simulink library "monroe_library"  (R2012b)
settings: Solver=ode45  StartTime=0.0  StopTime=10.0  RelTol=1e-3
values from neighbouring files (symbols this model uses):
  input_bit_width = ', num2str(input_bit_width))    [fft_direct_draw.m]
undefined symbols (not defined in the file or in its folder): gcbh, xlBlockLoadCallback
libraries: xbsIndex_r4 x1880, monroe_library x159, casper_library x13, xps_library x1
(part 41 of 43)

== system monroe_library/unscr_tail/mirror_spectrum/Subsystem ==
  In1 : Inport
  In3 : Inport  Port=2
  In4 : Inport  Port=3
  Delay11 : S-Function  LoadFcn=xlBlockLoadCallback(gcbh);  FunctionName=sysgen  Parameters=ptable_  EnableBusSupport=off  mask(Xilinx Delay Block){infoedit=Hardware notes: A delay line is a chain, each link of which is an SRL16 followed by a flip-flop., en_sgadvanced=, en=off, latency=1, dbl_ovrd_sgadvanced=, dbl_ovrd=off, reg_retiming_sgadvanced=, reg_retiming=off, xl_use_area_sgadvanced=, xl_use_area=off, xl_area=[0,0,0,0,0,0,0], has_advanced_control=0, sggui_pos=-1,-1,-1,-1, block_type=delay, block_version=, sg_icon_stat=25,28,1,1,white,blue,0,07b98262,right,,[ ],[ ], sg_mask_display=|, sg_list_contents=, sg_blockgui_xml=}
      mask sg_mask_display=|
      | fprintf('','COMMENT: begin icon graphics');
      | patch([0 25 25 0 0 ],[0 0 28 28 0 ],[0.77 0.82 0.91 ]);
      | plot([0 25 25 0 0 ],[0 0 28 28 0 ]);
      | patch([5.325 9.66 12.66 15.66 18.66 12.66 8.325 5.325 ],[17.33 17.33 20.33 17.33 20.33 20.33 20.33 17.33 ],[1 1 1 ]);
      | patch([8.325 12.66 9.66 5.325 8.325 ],[14.33 14.33 17.33 17.33 14.33 ],[0.931 0.946 0.973 ]);
      | patch([5.325 9.66 12.66 8.325 5.325 ],[11.33 11.33 14.33 14.33 11.33 ],[1 1 1 ]);
      | patch([8.325 18.66 15.66 12.66 9.66 5.325 8.325 ],[8.33 8.33 11.33 8.33 11.33 11.33 8.33 ],[0.931 0.946 0.973 ]);
      | fprintf('','COMMENT: end icon graphics');
      | fprintf('','COMMENT: begin icon text');
      |
      |
      | color('black');disp('z^{-1}','texmode','on');
      | fprintf('','COMMENT: end icon text');
      mask prompts: infoedit ""; en_sgadvanced ""; en "Provide enable port"; dbl_ovrd_sgadvanced ""; dbl_ovrd "Override with doubles"; reg_retiming_sgadvanced ""; reg_retiming "Implement using behavioral HDL."; xl_use_area_sgadvanced ""; xl_use_area "Define FPGA area for resource estimation"; xl_area "FPGA area [slices, FFs, BRAMs, LUTs, IOBs, emb. mults, TBUFs]"; has_advanced_control ""; sggui_pos ""; block_type ""; block_version ""; sg_icon_stat ""; sg_mask_display ""; sg_list_contents ""; sg_blockgui_xml ""
      mask help: Hardware notes: A delay line is a chain, each link of which is an SRL16 followed by a flip-flop.
      mask init: same as monroe_library/counter_limited_fast/Delay1
      settings: CopyFcn=xlBlockMoveCallback(gcbh);  DeleteFcn=xlDestroyGui(gcbh);  ModelCloseFcn=xlDestroyGui(gcbh);  PreSaveFcn=xlBlockPreSaveCallback(gcbh);  PostSaveFcn=xlBlockPostSaveCallback(gcbh);  DestroyFcn=xlDestroyGui(gcbh);  OpenFcn=xlOpenGui(gcbh, 'delay_gui.xml', @xlmagicenablement, -1)  CloseFcn=xlDestroyGui(gcbh);  MoveFcn=xlBlockMoveCallback(gcbh);
      mask Help: eval('');xlDoc('-book','sysgen','-topic','Delay');
      mask Display:
      | fprintf('','COMMENT: begin icon graphics');
      | patch([0 25 25 0 0 ],[0 0 28 28 0 ],[0.77 0.82 0.91 ]);
      | plot([0 25 25 0 0 ],[0 0 28 28 0 ]);
      | patch([5.325 9.66 12.66 15.66 18.66 12.66 8.325 5.325 ],[17.33 17.33 20.33 17.33 20.33 20.33 20.33 17.33 ],[1 1 1 ]);
      | patch([8.325 12.66 9.66 5.325 8.325 ],[14.33 14.33 17.33 17.33 14.33 ],[0.931 0.946 0.973 ]);
      | patch([5.325 9.66 12.66 8.325 5.325 ],[11.33 11.33 14.33 14.33 11.33 ],[1 1 1 ]);
      | patch([8.325 18.66 15.66 12.66 9.66 5.325 8.325 ],[8.33 8.33 11.33 8.33 11.33 11.33 8.33 ],[0.931 0.946 0.973 ]);
      | fprintf('','COMMENT: end icon graphics');
      | fprintf('','COMMENT: begin icon text');
      | 
      | 
      | color('black');disp('z^{-1}','texmode','on');
      | fprintf('','COMMENT: end icon text');
  Delay7 : xbsIndex_r4/Delay  en=off  latency=1  dbl_ovrd=off  reg_retiming=off  block_type=delay
  Mux4 : S-Function  LoadFcn=xlBlockLoadCallback(gcbh);  FunctionName=sysgen  Parameters=ptable_  EnableBusSupport=off  mask(Xilinx Bus Multiplexer Block){inputs_sgadvanced=, inputs=2, en_sgadvanced=, en=off, latency=0, precision_sgadvanced=, precision=Full, arith_type_sgadvanced=, arith_type=Signed  (2's comp), n_bits=8, bin_pt=2, quantization_sgadvanced=, quantization=Truncate, overflow_sgadvanced=, overflow=Wrap, dbl_ovrd_sgadvanced=, dbl_ovrd=off, xl_use_area_sgadvanced=, xl_use_area=off, xl_area=[0,0,0,0,0,0,0], infoedit=, has_advanced_control=0, sggui_pos=-1,-1,-1,-1, block_type=mux, block_version=, sg_icon_stat=45,104,3,1,white,blue,3,eb98d690,right,,[ ],[ ], sg_mask_display=|, sg_list_contents=, sg_blockgui_xml=}
      mask sg_mask_display=|
      | fprintf('','COMMENT: begin icon graphics');
      | patch([0 45 45 0 0 ],[0 14.8571 89.1429 104 0 ],[0.77 0.82 0.91 ]);
      | plot([0 45 45 0 0 ],[0 14.8571 89.1429 104 0 ]);
      | patch([8.65 17.32 23.32 29.32 35.32 23.32 14.65 8.65 ],[58.66 58.66 64.66 58.66 64.66 64.66 64.66 58.66 ],[1 1 1 ]);
      | patch([14.65 23.32 17.32 8.65 14.65 ],[52.66 52.66 58.66 58.66 52.66 ],[0.931 0.946 0.973 ]);
      | patch([8.65 17.32 23.32 14.65 8.65 ],[46.66 46.66 52.66 52.66 46.66 ],[1 1 1 ]);
      | patch([14.65 35.32 29.32 23.32 17.32 8.65 14.65 ],[40.66 40.66 46.66 40.66 46.66 46.66 40.66 ],[0.931 0.946 0.973 ]);
      | fprintf('','COMMENT: end icon graphics');
      | fprintf('','COMMENT: begin icon text');
      | color('black');port_label('input',1,'sel');
      | color('black');port_label('input',2,'d0');
      | color('black');port_label('input',3,'d1');
      |
      | color('black');disp('\bf{}','texmode','on');
      | fprintf('','COMMENT: end icon text');
      mask prompts: inputs_sgadvanced ""; inputs "Number of inputs"; en_sgadvanced ""; en "Provide enable port"; precision_sgadvanced ""; arith_type_sgadvanced ""; arith_type "Output type"; n_bits "Number of bits"; bin_pt "Binary point"; quantization_sgadvanced ""; overflow_sgadvanced ""; dbl_ovrd_sgadvanced ""; dbl_ovrd "Override with doubles"; xl_use_area_sgadvanced ""; xl_use_area "Define FPGA area for resource estimation"; xl_area "FPGA area [slices, FFs, BRAMs, LUTs, IOBs, emb. mults, TBUFs]"; infoedit ""; has_advanced_control ""; sggui_pos ""; block_type ""; block_version ""; sg_icon_stat ""; sg_mask_display ""; sg_list_contents ""; sg_blockgui_xml ""
      mask help: Xilinx Bus Multiplexer
      mask init:
      | try
      |   tmp_gcb = gcb;
      |   tmp_gcbh = gcbh;
      |   if (strcmp('SysGenIndex',get_param(bdroot(tmp_gcbh),'tag')) && ~isempty(regexp(bdroot(tmp_gcb), '^xbs', 'once')))
      |     return;
      |   end;
      |   xlMungeMaskParams;
      |   block_config = 'sysgen_blockset:Mux_config';
      | 
      |   block_type='mux';
      | 
      |   serialized_declarations = '{''arith_type''=>''Int'',''bin_pt''=>''Int'',''dbl_ovrd''=>''Int'',''en''=>''Int'',''inputs''=>''Int'',''latency''=>''Int'',''n_bits''=>''Int'',''overflow''=>''Int'',''period''=>''Double'',''precision''=>''Int'',''quantization''=>''Int'',''sim_engine''=>''Int'',''sysgen_root''=>''String'',''block_type''=>''String''}';
      |   xlmux_init();
      |   ptable_ = xlblockprep(get_param(tmp_gcb, 'MaskWSVariables'));
      |   try
      |     xlBlockMoveCallback(tmp_gcbh);
      |   catch 
      |      clear global xl_updateicon_recursion_guard;
      |   end;
      | catch
      |   global dbgsysgen;
      |   if(~isempty(dbgsysgen) && dbgsysgen)
      |     e = regexprep(lasterr, '\n', '\nError: ');
      |     disp(['Error: While running MaskInit code on block ' tmp_gcb ': ' e]);
      |     error(e);
      |   end
      | end
      settings: CopyFcn=xlBlockMoveCallback(gcbh);  DeleteFcn=xlDestroyGui(gcbh);  ModelCloseFcn=xlDestroyGui(gcbh);  PreSaveFcn=xlBlockPreSaveCallback(gcbh);  PostSaveFcn=xlBlockPostSaveCallback(gcbh);  DestroyFcn=xlDestroyGui(gcbh);  OpenFcn=xlOpenGui(gcbh, 'mux_gui.xml', @muxenablement, -1)  CloseFcn=xlDestroyGui(gcbh);  MoveFcn=xlBlockMoveCallback(gcbh);
      mask Help: eval('');xlDoc('-book','sysgen','-topic','Mux');
      mask TypeOptions inputs: 2 | 3 | 4 | 5 | 6 | 7 | 8 | 9 | 10 | 11 | 12 | 13 | 14 | 15 | 16 | 17 | 18 | 19 | 20 | 21 | 22 | 23 | 24 | 25 | 26 | 27 | 28 | 29 | 30 | 31 | 32
      mask TypeOptions precision: Full | User Defined
      mask TypeOptions arith_type: Signed  (2's comp) | Unsigned
      mask TypeOptions quantization: Truncate | Round  (unbiased: +/- Inf)
      mask TypeOptions overflow: Wrap | Saturate | Flag as error
      mask Display:
      | fprintf('','COMMENT: begin icon graphics');
      | patch([0 45 45 0 0 ],[0 14.8571 89.1429 104 0 ],[0.77 0.82 0.91 ]);
      | plot([0 45 45 0 0 ],[0 14.8571 89.1429 104 0 ]);
      | patch([8.65 17.32 23.32 29.32 35.32 23.32 14.65 8.65 ],[58.66 58.66 64.66 58.66 64.66 64.66 64.66 58.66 ],[1 1 1 ]);
      | patch([14.65 23.32 17.32 8.65 14.65 ],[52.66 52.66 58.66 58.66 52.66 ],[0.931 0.946 0.973 ]);
      | patch([8.65 17.32 23.32 14.65 8.65 ],[46.66 46.66 52.66 52.66 46.66 ],[1 1 1 ]);
      | patch([14.65 35.32 29.32 23.32 17.32 8.65 14.65 ],[40.66 40.66 46.66 40.66 46.66 46.66 40.66 ],[0.931 0.946 0.973 ]);
      | fprintf('','COMMENT: end icon graphics');
      | fprintf('','COMMENT: begin icon text');
      | color('black');port_label('input',1,'sel');
      | color('black');port_label('input',2,'d0');
      | color('black');port_label('input',3,'d1');
      | 
      | color('black');disp('\bf{}','texmode','on');
      | fprintf('','COMMENT: end icon text');
  Mux5 : S-Function  LoadFcn=xlBlockLoadCallback(gcbh);  FunctionName=sysgen  Parameters=ptable_  EnableBusSupport=off  mask(Xilinx Bus Multiplexer Block){inputs_sgadvanced=, inputs=2, en_sgadvanced=, en=off, latency=0, precision_sgadvanced=, precision=Full, arith_type_sgadvanced=, arith_type=Signed  (2's comp), n_bits=8, bin_pt=2, quantization_sgadvanced=, quantization=Truncate, overflow_sgadvanced=, overflow=Wrap, dbl_ovrd_sgadvanced=, dbl_ovrd=off, xl_use_area_sgadvanced=, xl_use_area=off, xl_area=[0,0,0,0,0,0,0], infoedit=, has_advanced_control=0, sggui_pos=-1,-1,-1,-1, block_type=mux, block_version=, sg_icon_stat=45,104,3,1,white,blue,3,eb98d690,right,,[ ],[ ], sg_mask_display=|, sg_list_contents=, sg_blockgui_xml=}
      mask sg_mask_display=|
      | fprintf('','COMMENT: begin icon graphics');
      | patch([0 45 45 0 0 ],[0 14.8571 89.1429 104 0 ],[0.77 0.82 0.91 ]);
      | plot([0 45 45 0 0 ],[0 14.8571 89.1429 104 0 ]);
      | patch([8.65 17.32 23.32 29.32 35.32 23.32 14.65 8.65 ],[58.66 58.66 64.66 58.66 64.66 64.66 64.66 58.66 ],[1 1 1 ]);
      | patch([14.65 23.32 17.32 8.65 14.65 ],[52.66 52.66 58.66 58.66 52.66 ],[0.931 0.946 0.973 ]);
      | patch([8.65 17.32 23.32 14.65 8.65 ],[46.66 46.66 52.66 52.66 46.66 ],[1 1 1 ]);
      | patch([14.65 35.32 29.32 23.32 17.32 8.65 14.65 ],[40.66 40.66 46.66 40.66 46.66 46.66 40.66 ],[0.931 0.946 0.973 ]);
      | fprintf('','COMMENT: end icon graphics');
      | fprintf('','COMMENT: begin icon text');
      | color('black');port_label('input',1,'sel');
      | color('black');port_label('input',2,'d0');
      | color('black');port_label('input',3,'d1');
      |
      | color('black');disp('\bf{}','texmode','on');
      | fprintf('','COMMENT: end icon text');
      mask prompts: inputs_sgadvanced ""; inputs "Number of inputs"; en_sgadvanced ""; en "Provide enable port"; precision_sgadvanced ""; arith_type_sgadvanced ""; arith_type "Output type"; n_bits "Number of bits"; bin_pt "Binary point"; quantization_sgadvanced ""; overflow_sgadvanced ""; dbl_ovrd_sgadvanced ""; dbl_ovrd "Override with doubles"; xl_use_area_sgadvanced ""; xl_use_area "Define FPGA area for resource estimation"; xl_area "FPGA area [slices, FFs, BRAMs, LUTs, IOBs, emb. mults, TBUFs]"; infoedit ""; has_advanced_control ""; sggui_pos ""; block_type ""; block_version ""; sg_icon_stat ""; sg_mask_display ""; sg_list_contents ""; sg_blockgui_xml ""
      mask help: Xilinx Bus Multiplexer
      mask init: same as monroe_library/unscr_tail/mirror_spectrum/Subsystem/Mux4
      settings: CopyFcn=xlBlockMoveCallback(gcbh);  DeleteFcn=xlDestroyGui(gcbh);  ModelCloseFcn=xlDestroyGui(gcbh);  PreSaveFcn=xlBlockPreSaveCallback(gcbh);  PostSaveFcn=xlBlockPostSaveCallback(gcbh);  DestroyFcn=xlDestroyGui(gcbh);  OpenFcn=xlOpenGui(gcbh, 'mux_gui.xml', @muxenablement, -1)  CloseFcn=xlDestroyGui(gcbh);  MoveFcn=xlBlockMoveCallback(gcbh);
      mask Help: eval('');xlDoc('-book','sysgen','-topic','Mux');
      mask TypeOptions inputs: 2 | 3 | 4 | 5 | 6 | 7 | 8 | 9 | 10 | 11 | 12 | 13 | 14 | 15 | 16 | 17 | 18 | 19 | 20 | 21 | 22 | 23 | 24 | 25 | 26 | 27 | 28 | 29 | 30 | 31 | 32
      mask TypeOptions precision: Full | User Defined
      mask TypeOptions arith_type: Signed  (2's comp) | Unsigned
      mask TypeOptions quantization: Truncate | Round  (unbiased: +/- Inf)
      mask TypeOptions overflow: Wrap | Saturate | Flag as error
      mask Display:
      | fprintf('','COMMENT: begin icon graphics');
      | patch([0 45 45 0 0 ],[0 14.8571 89.1429 104 0 ],[0.77 0.82 0.91 ]);
      | plot([0 45 45 0 0 ],[0 14.8571 89.1429 104 0 ]);
      | patch([8.65 17.32 23.32 29.32 35.32 23.32 14.65 8.65 ],[58.66 58.66 64.66 58.66 64.66 64.66 64.66 58.66 ],[1 1 1 ]);
      | patch([14.65 23.32 17.32 8.65 14.65 ],[52.66 52.66 58.66 58.66 52.66 ],[0.931 0.946 0.973 ]);
      | patch([8.65 17.32 23.32 14.65 8.65 ],[46.66 46.66 52.66 52.66 46.66 ],[1 1 1 ]);
      | patch([14.65 35.32 29.32 23.32 17.32 8.65 14.65 ],[40.66 40.66 46.66 40.66 46.66 46.66 40.66 ],[0.931 0.946 0.973 ]);
      | fprintf('','COMMENT: end icon graphics');
      | fprintf('','COMMENT: begin icon text');
      | color('black');port_label('input',1,'sel');
      | color('black');port_label('input',2,'d0');
      | color('black');port_label('input',3,'d1');
      | 
      | color('black');disp('\bf{}','texmode','on');
      | fprintf('','COMMENT: end icon text');
  cram5 : Subsystem
  uncram5 : monroe_library/unscr_tail/mirror_spectrum/uncram1  SystemSampleTime=-1
  uncram6 : Subsystem
  Out1 : Outport
  wires:
  uncram5/1 -> Mux4/2
  uncram6/1(out0) -> Mux4/3
  uncram5/2 -> Mux5/2
  uncram6/2(out1) -> Mux5/3
  Delay11/1 -> Mux4/1
  Delay7/1 -> Mux5/1
  Mux5/1 -> cram5/2(in1)
  Mux4/1 -> cram5/1(in0)
  In1/1 -> Delay11/1, Delay7/1
  cram5/1(out) -> Out1/1
  In3/1 -> uncram5/1
  In4/1 -> uncram6/1(in)

== system monroe_library/unscr_tail/mirror_spectrum/Subsystem1 ==
  In1 : Inport
  In3 : Inport  Port=2
  In4 : Inport  Port=3
  Delay11 : S-Function  LoadFcn=xlBlockLoadCallback(gcbh);  FunctionName=sysgen  Parameters=ptable_  EnableBusSupport=off  mask(Xilinx Delay Block){infoedit=Hardware notes: A delay line is a chain, each link of which is an SRL16 followed by a flip-flop., en_sgadvanced=, en=off, latency=1, dbl_ovrd_sgadvanced=, dbl_ovrd=off, reg_retiming_sgadvanced=, reg_retiming=off, xl_use_area_sgadvanced=, xl_use_area=off, xl_area=[0,0,0,0,0,0,0], has_advanced_control=0, sggui_pos=-1,-1,-1,-1, block_type=delay, block_version=, sg_icon_stat=25,28,1,1,white,blue,0,07b98262,right,,[ ],[ ], sg_mask_display=|, sg_list_contents=, sg_blockgui_xml=}
      mask sg_mask_display=|
      | fprintf('','COMMENT: begin icon graphics');
      | patch([0 25 25 0 0 ],[0 0 28 28 0 ],[0.77 0.82 0.91 ]);
      | plot([0 25 25 0 0 ],[0 0 28 28 0 ]);
      | patch([5.325 9.66 12.66 15.66 18.66 12.66 8.325 5.325 ],[17.33 17.33 20.33 17.33 20.33 20.33 20.33 17.33 ],[1 1 1 ]);
      | patch([8.325 12.66 9.66 5.325 8.325 ],[14.33 14.33 17.33 17.33 14.33 ],[0.931 0.946 0.973 ]);
      | patch([5.325 9.66 12.66 8.325 5.325 ],[11.33 11.33 14.33 14.33 11.33 ],[1 1 1 ]);
      | patch([8.325 18.66 15.66 12.66 9.66 5.325 8.325 ],[8.33 8.33 11.33 8.33 11.33 11.33 8.33 ],[0.931 0.946 0.973 ]);
      | fprintf('','COMMENT: end icon graphics');
      | fprintf('','COMMENT: begin icon text');
      |
      |
      | color('black');disp('z^{-1}','texmode','on');
      | fprintf('','COMMENT: end icon text');
      mask prompts: infoedit ""; en_sgadvanced ""; en "Provide enable port"; dbl_ovrd_sgadvanced ""; dbl_ovrd "Override with doubles"; reg_retiming_sgadvanced ""; reg_retiming "Implement using behavioral HDL."; xl_use_area_sgadvanced ""; xl_use_area "Define FPGA area for resource estimation"; xl_area "FPGA area [slices, FFs, BRAMs, LUTs, IOBs, emb. mults, TBUFs]"; has_advanced_control ""; sggui_pos ""; block_type ""; block_version ""; sg_icon_stat ""; sg_mask_display ""; sg_list_contents ""; sg_blockgui_xml ""
      mask help: Hardware notes: A delay line is a chain, each link of which is an SRL16 followed by a flip-flop.
      mask init: same as monroe_library/counter_limited_fast/Delay1
      settings: CopyFcn=xlBlockMoveCallback(gcbh);  DeleteFcn=xlDestroyGui(gcbh);  ModelCloseFcn=xlDestroyGui(gcbh);  PreSaveFcn=xlBlockPreSaveCallback(gcbh);  PostSaveFcn=xlBlockPostSaveCallback(gcbh);  DestroyFcn=xlDestroyGui(gcbh);  OpenFcn=xlOpenGui(gcbh, 'delay_gui.xml', @xlmagicenablement, -1)  CloseFcn=xlDestroyGui(gcbh);  MoveFcn=xlBlockMoveCallback(gcbh);
      mask Help: eval('');xlDoc('-book','sysgen','-topic','Delay');
      mask Display:
      | fprintf('','COMMENT: begin icon graphics');
      | patch([0 25 25 0 0 ],[0 0 28 28 0 ],[0.77 0.82 0.91 ]);
      | plot([0 25 25 0 0 ],[0 0 28 28 0 ]);
      | patch([5.325 9.66 12.66 15.66 18.66 12.66 8.325 5.325 ],[17.33 17.33 20.33 17.33 20.33 20.33 20.33 17.33 ],[1 1 1 ]);
      | patch([8.325 12.66 9.66 5.325 8.325 ],[14.33 14.33 17.33 17.33 14.33 ],[0.931 0.946 0.973 ]);
      | patch([5.325 9.66 12.66 8.325 5.325 ],[11.33 11.33 14.33 14.33 11.33 ],[1 1 1 ]);
      | patch([8.325 18.66 15.66 12.66 9.66 5.325 8.325 ],[8.33 8.33 11.33 8.33 11.33 11.33 8.33 ],[0.931 0.946 0.973 ]);
      | fprintf('','COMMENT: end icon graphics');
      | fprintf('','COMMENT: begin icon text');
      | 
      | 
      | color('black');disp('z^{-1}','texmode','on');
      | fprintf('','COMMENT: end icon text');
  Delay7 : xbsIndex_r4/Delay  en=off  latency=1  dbl_ovrd=off  reg_retiming=off  block_type=delay
  Mux4 : S-Function  LoadFcn=xlBlockLoadCallback(gcbh);  FunctionName=sysgen  Parameters=ptable_  EnableBusSupport=off  mask(Xilinx Bus Multiplexer Block){inputs_sgadvanced=, inputs=2, en_sgadvanced=, en=off, latency=0, precision_sgadvanced=, precision=Full, arith_type_sgadvanced=, arith_type=Signed  (2's comp), n_bits=8, bin_pt=2, quantization_sgadvanced=, quantization=Truncate, overflow_sgadvanced=, overflow=Wrap, dbl_ovrd_sgadvanced=, dbl_ovrd=off, xl_use_area_sgadvanced=, xl_use_area=off, xl_area=[0,0,0,0,0,0,0], infoedit=, has_advanced_control=0, sggui_pos=-1,-1,-1,-1, block_type=mux, block_version=, sg_icon_stat=45,104,3,1,white,blue,3,eb98d690,right,,[ ],[ ], sg_mask_display=|, sg_list_contents=, sg_blockgui_xml=}
      mask sg_mask_display=|
      | fprintf('','COMMENT: begin icon graphics');
      | patch([0 45 45 0 0 ],[0 14.8571 89.1429 104 0 ],[0.77 0.82 0.91 ]);
      | plot([0 45 45 0 0 ],[0 14.8571 89.1429 104 0 ]);
      | patch([8.65 17.32 23.32 29.32 35.32 23.32 14.65 8.65 ],[58.66 58.66 64.66 58.66 64.66 64.66 64.66 58.66 ],[1 1 1 ]);
      | patch([14.65 23.32 17.32 8.65 14.65 ],[52.66 52.66 58.66 58.66 52.66 ],[0.931 0.946 0.973 ]);
      | patch([8.65 17.32 23.32 14.65 8.65 ],[46.66 46.66 52.66 52.66 46.66 ],[1 1 1 ]);
      | patch([14.65 35.32 29.32 23.32 17.32 8.65 14.65 ],[40.66 40.66 46.66 40.66 46.66 46.66 40.66 ],[0.931 0.946 0.973 ]);
      | fprintf('','COMMENT: end icon graphics');
      | fprintf('','COMMENT: begin icon text');
      | color('black');port_label('input',1,'sel');
      | color('black');port_label('input',2,'d0');
      | color('black');port_label('input',3,'d1');
      |
      | color('black');disp('\bf{}','texmode','on');
      | fprintf('','COMMENT: end icon text');
      mask prompts: inputs_sgadvanced ""; inputs "Number of inputs"; en_sgadvanced ""; en "Provide enable port"; precision_sgadvanced ""; arith_type_sgadvanced ""; arith_type "Output type"; n_bits "Number of bits"; bin_pt "Binary point"; quantization_sgadvanced ""; overflow_sgadvanced ""; dbl_ovrd_sgadvanced ""; dbl_ovrd "Override with doubles"; xl_use_area_sgadvanced ""; xl_use_area "Define FPGA area for resource estimation"; xl_area "FPGA area [slices, FFs, BRAMs, LUTs, IOBs, emb. mults, TBUFs]"; infoedit ""; has_advanced_control ""; sggui_pos ""; block_type ""; block_version ""; sg_icon_stat ""; sg_mask_display ""; sg_list_contents ""; sg_blockgui_xml ""
      mask help: Xilinx Bus Multiplexer
      mask init: same as monroe_library/unscr_tail/mirror_spectrum/Subsystem/Mux4
      settings: CopyFcn=xlBlockMoveCallback(gcbh);  DeleteFcn=xlDestroyGui(gcbh);  ModelCloseFcn=xlDestroyGui(gcbh);  PreSaveFcn=xlBlockPreSaveCallback(gcbh);  PostSaveFcn=xlBlockPostSaveCallback(gcbh);  DestroyFcn=xlDestroyGui(gcbh);  OpenFcn=xlOpenGui(gcbh, 'mux_gui.xml', @muxenablement, -1)  CloseFcn=xlDestroyGui(gcbh);  MoveFcn=xlBlockMoveCallback(gcbh);
      mask Help: eval('');xlDoc('-book','sysgen','-topic','Mux');
      mask TypeOptions inputs: 2 | 3 | 4 | 5 | 6 | 7 | 8 | 9 | 10 | 11 | 12 | 13 | 14 | 15 | 16 | 17 | 18 | 19 | 20 | 21 | 22 | 23 | 24 | 25 | 26 | 27 | 28 | 29 | 30 | 31 | 32
      mask TypeOptions precision: Full | User Defined
      mask TypeOptions arith_type: Signed  (2's comp) | Unsigned
      mask TypeOptions quantization: Truncate | Round  (unbiased: +/- Inf)
      mask TypeOptions overflow: Wrap | Saturate | Flag as error
      mask Display:
      | fprintf('','COMMENT: begin icon graphics');
      | patch([0 45 45 0 0 ],[0 14.8571 89.1429 104 0 ],[0.77 0.82 0.91 ]);
      | plot([0 45 45 0 0 ],[0 14.8571 89.1429 104 0 ]);
      | patch([8.65 17.32 23.32 29.32 35.32 23.32 14.65 8.65 ],[58.66 58.66 64.66 58.66 64.66 64.66 64.66 58.66 ],[1 1 1 ]);
      | patch([14.65 23.32 17.32 8.65 14.65 ],[52.66 52.66 58.66 58.66 52.66 ],[0.931 0.946 0.973 ]);
      | patch([8.65 17.32 23.32 14.65 8.65 ],[46.66 46.66 52.66 52.66 46.66 ],[1 1 1 ]);
      | patch([14.65 35.32 29.32 23.32 17.32 8.65 14.65 ],[40.66 40.66 46.66 40.66 46.66 46.66 40.66 ],[0.931 0.946 0.973 ]);
      | fprintf('','COMMENT: end icon graphics');
      | fprintf('','COMMENT: begin icon text');
      | color('black');port_label('input',1,'sel');
      | color('black');port_label('input',2,'d0');
      | color('black');port_label('input',3,'d1');
      | 
      | color('black');disp('\bf{}','texmode','on');
      | fprintf('','COMMENT: end icon text');
  Mux5 : S-Function  LoadFcn=xlBlockLoadCallback(gcbh);  FunctionName=sysgen  Parameters=ptable_  EnableBusSupport=off  mask(Xilinx Bus Multiplexer Block){inputs_sgadvanced=, inputs=2, en_sgadvanced=, en=off, latency=0, precision_sgadvanced=, precision=Full, arith_type_sgadvanced=, arith_type=Signed  (2's comp), n_bits=8, bin_pt=2, quantization_sgadvanced=, quantization=Truncate, overflow_sgadvanced=, overflow=Wrap, dbl_ovrd_sgadvanced=, dbl_ovrd=off, xl_use_area_sgadvanced=, xl_use_area=off, xl_area=[0,0,0,0,0,0,0], infoedit=, has_advanced_control=0, sggui_pos=-1,-1,-1,-1, block_type=mux, block_version=, sg_icon_stat=45,104,3,1,white,blue,3,eb98d690,right,,[ ],[ ], sg_mask_display=|, sg_list_contents=, sg_blockgui_xml=}
      mask sg_mask_display=|
      | fprintf('','COMMENT: begin icon graphics');
      | patch([0 45 45 0 0 ],[0 14.8571 89.1429 104 0 ],[0.77 0.82 0.91 ]);
      | plot([0 45 45 0 0 ],[0 14.8571 89.1429 104 0 ]);
      | patch([8.65 17.32 23.32 29.32 35.32 23.32 14.65 8.65 ],[58.66 58.66 64.66 58.66 64.66 64.66 64.66 58.66 ],[1 1 1 ]);
      | patch([14.65 23.32 17.32 8.65 14.65 ],[52.66 52.66 58.66 58.66 52.66 ],[0.931 0.946 0.973 ]);
      | patch([8.65 17.32 23.32 14.65 8.65 ],[46.66 46.66 52.66 52.66 46.66 ],[1 1 1 ]);
      | patch([14.65 35.32 29.32 23.32 17.32 8.65 14.65 ],[40.66 40.66 46.66 40.66 46.66 46.66 40.66 ],[0.931 0.946 0.973 ]);
      | fprintf('','COMMENT: end icon graphics');
      | fprintf('','COMMENT: begin icon text');
      | color('black');port_label('input',1,'sel');
      | color('black');port_label('input',2,'d0');
      | color('black');port_label('input',3,'d1');
      |
      | color('black');disp('\bf{}','texmode','on');
      | fprintf('','COMMENT: end icon text');
      mask prompts: inputs_sgadvanced ""; inputs "Number of inputs"; en_sgadvanced ""; en "Provide enable port"; precision_sgadvanced ""; arith_type_sgadvanced ""; arith_type "Output type"; n_bits "Number of bits"; bin_pt "Binary point"; quantization_sgadvanced ""; overflow_sgadvanced ""; dbl_ovrd_sgadvanced ""; dbl_ovrd "Override with doubles"; xl_use_area_sgadvanced ""; xl_use_area "Define FPGA area for resource estimation"; xl_area "FPGA area [slices, FFs, BRAMs, LUTs, IOBs, emb. mults, TBUFs]"; infoedit ""; has_advanced_control ""; sggui_pos ""; block_type ""; block_version ""; sg_icon_stat ""; sg_mask_display ""; sg_list_contents ""; sg_blockgui_xml ""
      mask help: Xilinx Bus Multiplexer
      mask init: same as monroe_library/unscr_tail/mirror_spectrum/Subsystem/Mux4
      settings: CopyFcn=xlBlockMoveCallback(gcbh);  DeleteFcn=xlDestroyGui(gcbh);  ModelCloseFcn=xlDestroyGui(gcbh);  PreSaveFcn=xlBlockPreSaveCallback(gcbh);  PostSaveFcn=xlBlockPostSaveCallback(gcbh);  DestroyFcn=xlDestroyGui(gcbh);  OpenFcn=xlOpenGui(gcbh, 'mux_gui.xml', @muxenablement, -1)  CloseFcn=xlDestroyGui(gcbh);  MoveFcn=xlBlockMoveCallback(gcbh);
      mask Help: eval('');xlDoc('-book','sysgen','-topic','Mux');
      mask TypeOptions inputs: 2 | 3 | 4 | 5 | 6 | 7 | 8 | 9 | 10 | 11 | 12 | 13 | 14 | 15 | 16 | 17 | 18 | 19 | 20 | 21 | 22 | 23 | 24 | 25 | 26 | 27 | 28 | 29 | 30 | 31 | 32
      mask TypeOptions precision: Full | User Defined
      mask TypeOptions arith_type: Signed  (2's comp) | Unsigned
      mask TypeOptions quantization: Truncate | Round  (unbiased: +/- Inf)
      mask TypeOptions overflow: Wrap | Saturate | Flag as error
      mask Display:
      | fprintf('','COMMENT: begin icon graphics');
      | patch([0 45 45 0 0 ],[0 14.8571 89.1429 104 0 ],[0.77 0.82 0.91 ]);
      | plot([0 45 45 0 0 ],[0 14.8571 89.1429 104 0 ]);
      | patch([8.65 17.32 23.32 29.32 35.32 23.32 14.65 8.65 ],[58.66 58.66 64.66 58.66 64.66 64.66 64.66 58.66 ],[1 1 1 ]);
      | patch([14.65 23.32 17.32 8.65 14.65 ],[52.66 52.66 58.66 58.66 52.66 ],[0.931 0.946 0.973 ]);
      | patch([8.65 17.32 23.32 14.65 8.65 ],[46.66 46.66 52.66 52.66 46.66 ],[1 1 1 ]);
      | patch([14.65 35.32 29.32 23.32 17.32 8.65 14.65 ],[40.66 40.66 46.66 40.66 46.66 46.66 40.66 ],[0.931 0.946 0.973 ]);
      | fprintf('','COMMENT: end icon graphics');
      | fprintf('','COMMENT: begin icon text');
      | color('black');port_label('input',1,'sel');
      | color('black');port_label('input',2,'d0');
      | color('black');port_label('input',3,'d1');
      | 
      | color('black');disp('\bf{}','texmode','on');
      | fprintf('','COMMENT: end icon text');
  cram5 : Subsystem
  uncram5 : monroe_library/unscr_tail/mirror_spectrum/uncram1  SystemSampleTime=-1
  uncram6 : Subsystem
  Out1 : Outport
  wires:
  In4/1 -> uncram6/1(in)
  In3/1 -> uncram5/1
  cram5/1(out) -> Out1/1
  In1/1 -> Delay7/1, Delay11/1
  Mux4/1 -> cram5/1(in0)
  Mux5/1 -> cram5/2(in1)
  Delay7/1 -> Mux5/1
  Delay11/1 -> Mux4/1
  uncram6/2(out1) -> Mux5/3
  uncram5/2 -> Mux5/2
  uncram6/1(out0) -> Mux4/3
  uncram5/1 -> Mux4/2

== system monroe_library/unscr_tail/mirror_spectrum/Subsystem2 ==
  In1 : Inport
  In3 : Inport  Port=2
  In4 : Inport  Port=3
  Delay11 : S-Function  LoadFcn=xlBlockLoadCallback(gcbh);  FunctionName=sysgen  Parameters=ptable_  EnableBusSupport=off  mask(Xilinx Delay Block){infoedit=Hardware notes: A delay line is a chain, each link of which is an SRL16 followed by a flip-flop., en_sgadvanced=, en=off, latency=1, dbl_ovrd_sgadvanced=, dbl_ovrd=off, reg_retiming_sgadvanced=, reg_retiming=off, xl_use_area_sgadvanced=, xl_use_area=off, xl_area=[0,0,0,0,0,0,0], has_advanced_control=0, sggui_pos=-1,-1,-1,-1, block_type=delay, block_version=, sg_icon_stat=25,28,1,1,white,blue,0,07b98262,right,,[ ],[ ], sg_mask_display=|, sg_list_contents=, sg_blockgui_xml=}
      mask sg_mask_display=|
      | fprintf('','COMMENT: begin icon graphics');
      | patch([0 25 25 0 0 ],[0 0 28 28 0 ],[0.77 0.82 0.91 ]);
      | plot([0 25 25 0 0 ],[0 0 28 28 0 ]);
      | patch([5.325 9.66 12.66 15.66 18.66 12.66 8.325 5.325 ],[17.33 17.33 20.33 17.33 20.33 20.33 20.33 17.33 ],[1 1 1 ]);
      | patch([8.325 12.66 9.66 5.325 8.325 ],[14.33 14.33 17.33 17.33 14.33 ],[0.931 0.946 0.973 ]);
      | patch([5.325 9.66 12.66 8.325 5.325 ],[11.33 11.33 14.33 14.33 11.33 ],[1 1 1 ]);
      | patch([8.325 18.66 15.66 12.66 9.66 5.325 8.325 ],[8.33 8.33 11.33 8.33 11.33 11.33 8.33 ],[0.931 0.946 0.973 ]);
      | fprintf('','COMMENT: end icon graphics');
      | fprintf('','COMMENT: begin icon text');
      |
      |
      | color('black');disp('z^{-1}','texmode','on');
      | fprintf('','COMMENT: end icon text');
      mask prompts: infoedit ""; en_sgadvanced ""; en "Provide enable port"; dbl_ovrd_sgadvanced ""; dbl_ovrd "Override with doubles"; reg_retiming_sgadvanced ""; reg_retiming "Implement using behavioral HDL."; xl_use_area_sgadvanced ""; xl_use_area "Define FPGA area for resource estimation"; xl_area "FPGA area [slices, FFs, BRAMs, LUTs, IOBs, emb. mults, TBUFs]"; has_advanced_control ""; sggui_pos ""; block_type ""; block_version ""; sg_icon_stat ""; sg_mask_display ""; sg_list_contents ""; sg_blockgui_xml ""
      mask help: Hardware notes: A delay line is a chain, each link of which is an SRL16 followed by a flip-flop.
      mask init: same as monroe_library/counter_limited_fast/Delay1
      settings: CopyFcn=xlBlockMoveCallback(gcbh);  DeleteFcn=xlDestroyGui(gcbh);  ModelCloseFcn=xlDestroyGui(gcbh);  PreSaveFcn=xlBlockPreSaveCallback(gcbh);  PostSaveFcn=xlBlockPostSaveCallback(gcbh);  DestroyFcn=xlDestroyGui(gcbh);  OpenFcn=xlOpenGui(gcbh, 'delay_gui.xml', @xlmagicenablement, -1)  CloseFcn=xlDestroyGui(gcbh);  MoveFcn=xlBlockMoveCallback(gcbh);
      mask Help: eval('');xlDoc('-book','sysgen','-topic','Delay');
      mask Display:
      | fprintf('','COMMENT: begin icon graphics');
      | patch([0 25 25 0 0 ],[0 0 28 28 0 ],[0.77 0.82 0.91 ]);
      | plot([0 25 25 0 0 ],[0 0 28 28 0 ]);
      | patch([5.325 9.66 12.66 15.66 18.66 12.66 8.325 5.325 ],[17.33 17.33 20.33 17.33 20.33 20.33 20.33 17.33 ],[1 1 1 ]);
      | patch([8.325 12.66 9.66 5.325 8.325 ],[14.33 14.33 17.33 17.33 14.33 ],[0.931 0.946 0.973 ]);
      | patch([5.325 9.66 12.66 8.325 5.325 ],[11.33 11.33 14.33 14.33 11.33 ],[1 1 1 ]);
      | patch([8.325 18.66 15.66 12.66 9.66 5.325 8.325 ],[8.33 8.33 11.33 8.33 11.33 11.33 8.33 ],[0.931 0.946 0.973 ]);
      | fprintf('','COMMENT: end icon graphics');
      | fprintf('','COMMENT: begin icon text');
      | 
      | 
      | color('black');disp('z^{-1}','texmode','on');
      | fprintf('','COMMENT: end icon text');
  Delay7 : xbsIndex_r4/Delay  en=off  latency=1  dbl_ovrd=off  reg_retiming=off  block_type=delay
  Mux4 : S-Function  LoadFcn=xlBlockLoadCallback(gcbh);  FunctionName=sysgen  Parameters=ptable_  EnableBusSupport=off  mask(Xilinx Bus Multiplexer Block){inputs_sgadvanced=, inputs=2, en_sgadvanced=, en=off, latency=0, precision_sgadvanced=, precision=Full, arith_type_sgadvanced=, arith_type=Signed  (2's comp), n_bits=8, bin_pt=2, quantization_sgadvanced=, quantization=Truncate, overflow_sgadvanced=, overflow=Wrap, dbl_ovrd_sgadvanced=, dbl_ovrd=off, xl_use_area_sgadvanced=, xl_use_area=off, xl_area=[0,0,0,0,0,0,0], infoedit=, has_advanced_control=0, sggui_pos=-1,-1,-1,-1, block_type=mux, block_version=, sg_icon_stat=45,104,3,1,white,blue,3,eb98d690,right,,[ ],[ ], sg_mask_display=|, sg_list_contents=, sg_blockgui_xml=}
      mask sg_mask_display=|
      | fprintf('','COMMENT: begin icon graphics');
      | patch([0 45 45 0 0 ],[0 14.8571 89.1429 104 0 ],[0.77 0.82 0.91 ]);
      | plot([0 45 45 0 0 ],[0 14.8571 89.1429 104 0 ]);
      | patch([8.65 17.32 23.32 29.32 35.32 23.32 14.65 8.65 ],[58.66 58.66 64.66 58.66 64.66 64.66 64.66 58.66 ],[1 1 1 ]);
      | patch([14.65 23.32 17.32 8.65 14.65 ],[52.66 52.66 58.66 58.66 52.66 ],[0.931 0.946 0.973 ]);
      | patch([8.65 17.32 23.32 14.65 8.65 ],[46.66 46.66 52.66 52.66 46.66 ],[1 1 1 ]);
      | patch([14.65 35.32 29.32 23.32 17.32 8.65 14.65 ],[40.66 40.66 46.66 40.66 46.66 46.66 40.66 ],[0.931 0.946 0.973 ]);
      | fprintf('','COMMENT: end icon graphics');
      | fprintf('','COMMENT: begin icon text');
      | color('black');port_label('input',1,'sel');
      | color('black');port_label('input',2,'d0');
      | color('black');port_label('input',3,'d1');
      |
      | color('black');disp('\bf{}','texmode','on');
      | fprintf('','COMMENT: end icon text');
      mask prompts: inputs_sgadvanced ""; inputs "Number of inputs"; en_sgadvanced ""; en "Provide enable port"; precision_sgadvanced ""; arith_type_sgadvanced ""; arith_type "Output type"; n_bits "Number of bits"; bin_pt "Binary point"; quantization_sgadvanced ""; overflow_sgadvanced ""; dbl_ovrd_sgadvanced ""; dbl_ovrd "Override with doubles"; xl_use_area_sgadvanced ""; xl_use_area "Define FPGA area for resource estimation"; xl_area "FPGA area [slices, FFs, BRAMs, LUTs, IOBs, emb. mults, TBUFs]"; infoedit ""; has_advanced_control ""; sggui_pos ""; block_type ""; block_version ""; sg_icon_stat ""; sg_mask_display ""; sg_list_contents ""; sg_blockgui_xml ""
      mask help: Xilinx Bus Multiplexer
      mask init: same as monroe_library/unscr_tail/mirror_spectrum/Subsystem/Mux4
      settings: CopyFcn=xlBlockMoveCallback(gcbh);  DeleteFcn=xlDestroyGui(gcbh);  ModelCloseFcn=xlDestroyGui(gcbh);  PreSaveFcn=xlBlockPreSaveCallback(gcbh);  PostSaveFcn=xlBlockPostSaveCallback(gcbh);  DestroyFcn=xlDestroyGui(gcbh);  OpenFcn=xlOpenGui(gcbh, 'mux_gui.xml', @muxenablement, -1)  CloseFcn=xlDestroyGui(gcbh);  MoveFcn=xlBlockMoveCallback(gcbh);
      mask Help: eval('');xlDoc('-book','sysgen','-topic','Mux');
      mask TypeOptions inputs: 2 | 3 | 4 | 5 | 6 | 7 | 8 | 9 | 10 | 11 | 12 | 13 | 14 | 15 | 16 | 17 | 18 | 19 | 20 | 21 | 22 | 23 | 24 | 25 | 26 | 27 | 28 | 29 | 30 | 31 | 32
      mask TypeOptions precision: Full | User Defined
      mask TypeOptions arith_type: Signed  (2's comp) | Unsigned
      mask TypeOptions quantization: Truncate | Round  (unbiased: +/- Inf)
      mask TypeOptions overflow: Wrap | Saturate | Flag as error
      mask Display:
      | fprintf('','COMMENT: begin icon graphics');
      | patch([0 45 45 0 0 ],[0 14.8571 89.1429 104 0 ],[0.77 0.82 0.91 ]);
      | plot([0 45 45 0 0 ],[0 14.8571 89.1429 104 0 ]);
      | patch([8.65 17.32 23.32 29.32 35.32 23.32 14.65 8.65 ],[58.66 58.66 64.66 58.66 64.66 64.66 64.66 58.66 ],[1 1 1 ]);
      | patch([14.65 23.32 17.32 8.65 14.65 ],[52.66 52.66 58.66 58.66 52.66 ],[0.931 0.946 0.973 ]);
      | patch([8.65 17.32 23.32 14.65 8.65 ],[46.66 46.66 52.66 52.66 46.66 ],[1 1 1 ]);
      | patch([14.65 35.32 29.32 23.32 17.32 8.65 14.65 ],[40.66 40.66 46.66 40.66 46.66 46.66 40.66 ],[0.931 0.946 0.973 ]);
      | fprintf('','COMMENT: end icon graphics');
      | fprintf('','COMMENT: begin icon text');
      | color('black');port_label('input',1,'sel');
      | color('black');port_label('input',2,'d0');
      | color('black');port_label('input',3,'d1');
      | 
      | color('black');disp('\bf{}','texmode','on');
      | fprintf('','COMMENT: end icon text');
  Mux5 : S-Function  LoadFcn=xlBlockLoadCallback(gcbh);  FunctionName=sysgen  Parameters=ptable_  EnableBusSupport=off  mask(Xilinx Bus Multiplexer Block){inputs_sgadvanced=, inputs=2, en_sgadvanced=, en=off, latency=0, precision_sgadvanced=, precision=Full, arith_type_sgadvanced=, arith_type=Signed  (2's comp), n_bits=8, bin_pt=2, quantization_sgadvanced=, quantization=Truncate, overflow_sgadvanced=, overflow=Wrap, dbl_ovrd_sgadvanced=, dbl_ovrd=off, xl_use_area_sgadvanced=, xl_use_area=off, xl_area=[0,0,0,0,0,0,0], infoedit=, has_advanced_control=0, sggui_pos=-1,-1,-1,-1, block_type=mux, block_version=, sg_icon_stat=45,104,3,1,white,blue,3,eb98d690,right,,[ ],[ ], sg_mask_display=|, sg_list_contents=, sg_blockgui_xml=}
      mask sg_mask_display=|
      | fprintf('','COMMENT: begin icon graphics');
      | patch([0 45 45 0 0 ],[0 14.8571 89.1429 104 0 ],[0.77 0.82 0.91 ]);
      | plot([0 45 45 0 0 ],[0 14.8571 89.1429 104 0 ]);
      | patch([8.65 17.32 23.32 29.32 35.32 23.32 14.65 8.65 ],[58.66 58.66 64.66 58.66 64.66 64.66 64.66 58.66 ],[1 1 1 ]);
      | patch([14.65 23.32 17.32 8.65 14.65 ],[52.66 52.66 58.66 58.66 52.66 ],[0.931 0.946 0.973 ]);
      | patch([8.65 17.32 23.32 14.65 8.65 ],[46.66 46.66 52.66 52.66 46.66 ],[1 1 1 ]);
      | patch([14.65 35.32 29.32 23.32 17.32 8.65 14.65 ],[40.66 40.66 46.66 40.66 46.66 46.66 40.66 ],[0.931 0.946 0.973 ]);
      | fprintf('','COMMENT: end icon graphics');
      | fprintf('','COMMENT: begin icon text');
      | color('black');port_label('input',1,'sel');
      | color('black');port_label('input',2,'d0');
      | color('black');port_label('input',3,'d1');
      |
      | color('black');disp('\bf{}','texmode','on');
      | fprintf('','COMMENT: end icon text');
      mask prompts: inputs_sgadvanced ""; inputs "Number of inputs"; en_sgadvanced ""; en "Provide enable port"; precision_sgadvanced ""; arith_type_sgadvanced ""; arith_type "Output type"; n_bits "Number of bits"; bin_pt "Binary point"; quantization_sgadvanced ""; overflow_sgadvanced ""; dbl_ovrd_sgadvanced ""; dbl_ovrd "Override with doubles"; xl_use_area_sgadvanced ""; xl_use_area "Define FPGA area for resource estimation"; xl_area "FPGA area [slices, FFs, BRAMs, LUTs, IOBs, emb. mults, TBUFs]"; infoedit ""; has_advanced_control ""; sggui_pos ""; block_type ""; block_version ""; sg_icon_stat ""; sg_mask_display ""; sg_list_contents ""; sg_blockgui_xml ""
      mask help: Xilinx Bus Multiplexer
      mask init: same as monroe_library/unscr_tail/mirror_spectrum/Subsystem/Mux4
      settings: CopyFcn=xlBlockMoveCallback(gcbh);  DeleteFcn=xlDestroyGui(gcbh);  ModelCloseFcn=xlDestroyGui(gcbh);  PreSaveFcn=xlBlockPreSaveCallback(gcbh);  PostSaveFcn=xlBlockPostSaveCallback(gcbh);  DestroyFcn=xlDestroyGui(gcbh);  OpenFcn=xlOpenGui(gcbh, 'mux_gui.xml', @muxenablement, -1)  CloseFcn=xlDestroyGui(gcbh);  MoveFcn=xlBlockMoveCallback(gcbh);
      mask Help: eval('');xlDoc('-book','sysgen','-topic','Mux');
      mask TypeOptions inputs: 2 | 3 | 4 | 5 | 6 | 7 | 8 | 9 | 10 | 11 | 12 | 13 | 14 | 15 | 16 | 17 | 18 | 19 | 20 | 21 | 22 | 23 | 24 | 25 | 26 | 27 | 28 | 29 | 30 | 31 | 32
      mask TypeOptions precision: Full | User Defined
      mask TypeOptions arith_type: Signed  (2's comp) | Unsigned
      mask TypeOptions quantization: Truncate | Round  (unbiased: +/- Inf)
      mask TypeOptions overflow: Wrap | Saturate | Flag as error
      mask Display:
      | fprintf('','COMMENT: begin icon graphics');
      | patch([0 45 45 0 0 ],[0 14.8571 89.1429 104 0 ],[0.77 0.82 0.91 ]);
      | plot([0 45 45 0 0 ],[0 14.8571 89.1429 104 0 ]);
      | patch([8.65 17.32 23.32 29.32 35.32 23.32 14.65 8.65 ],[58.66 58.66 64.66 58.66 64.66 64.66 64.66 58.66 ],[1 1 1 ]);
      | patch([14.65 23.32 17.32 8.65 14.65 ],[52.66 52.66 58.66 58.66 52.66 ],[0.931 0.946 0.973 ]);
      | patch([8.65 17.32 23.32 14.65 8.65 ],[46.66 46.66 52.66 52.66 46.66 ],[1 1 1 ]);
      | patch([14.65 35.32 29.32 23.32 17.32 8.65 14.65 ],[40.66 40.66 46.66 40.66 46.66 46.66 40.66 ],[0.931 0.946 0.973 ]);
      | fprintf('','COMMENT: end icon graphics');
      | fprintf('','COMMENT: begin icon text');
      | color('black');port_label('input',1,'sel');
      | color('black');port_label('input',2,'d0');
      | color('black');port_label('input',3,'d1');
      | 
      | color('black');disp('\bf{}','texmode','on');
      | fprintf('','COMMENT: end icon text');
  cram5 : Subsystem
  uncram5 : monroe_library/unscr_tail/mirror_spectrum/uncram1  SystemSampleTime=-1
  uncram6 : Subsystem
  Out1 : Outport
  wires:
  uncram5/1 -> Mux4/2
  uncram6/1(out0) -> Mux4/3
  uncram5/2 -> Mux5/2
  uncram6/2(out1) -> Mux5/3
  Delay11/1 -> Mux4/1
  Delay7/1 -> Mux5/1
  Mux5/1 -> cram5/2(in1)
  Mux4/1 -> cram5/1(in0)
  In1/1 -> Delay11/1, Delay7/1
  cram5/1(out) -> Out1/1
  In3/1 -> uncram5/1
  In4/1 -> uncram6/1(in)
